simulink model "testBCIRobot3e_sim"  (Simulink 10.0)
settings: Solver=FixedStepDiscrete  StartTime=0.0  StopTime=10  FixedStep=0.002  MaxStep=0.02  RelTol=1e-3  AbsTol=1e-6
libraries: simulink_extras x1
settings Model: Creator=fwornle  LastModifiedBy=bhisma  ExtModeTrigDuration=5000  ExtModeLogAll=off
settings ConfigSet: Description=rtmc9s12target_R2008a
settings SolverCC: AutoScaleAbsTol=off
settings DataIOCC: SignalLoggingSaveFormat=ModelDataLogs  SaveOutput=off  SaveTime=off  SignalLoggingName=sigsOut
settings OptimizationCC: BlockReduction=off  BooleanDataType=off  ExpressionDepthLimit=2147483647  InitFltsAndDblsToZero=on
settings DebuggingCC: SaveWithParameterizedLinksMsg=none  SignalResolutionControl=TryResolveAllWithWarning  MultiTaskDSMMsg=warning  MultiTaskCondExecSysMsg=none  FcnCallInpInsideContextMsg=warning  StateNameClashWarn=warning
settings HardwareCC: ProdBitPerInt=16  ProdBitPerPointer=16  ProdBitPerSizeT=16  ProdBitPerPtrDiffT=16  ProdEndianess=BigEndian  ProdWordSize=16  ProdHWDeviceType=Motorola HC12  TargetHWDeviceType=32-bit Generic  ProdEqTarget=off
settings RTWCC: Description="Visual C/C++ Project Makefile only for the \"grt\" target"  GenerateMakefile=off  TemplateMakefile=grt_msvc.tmf
settings GRTTargetCC: TargetFcnLib=ansi_tfl_tmw.mat  GeneratePreprocessorConditionals=Disable all
settings ConfigComp: CovExternalEMLEnable=off

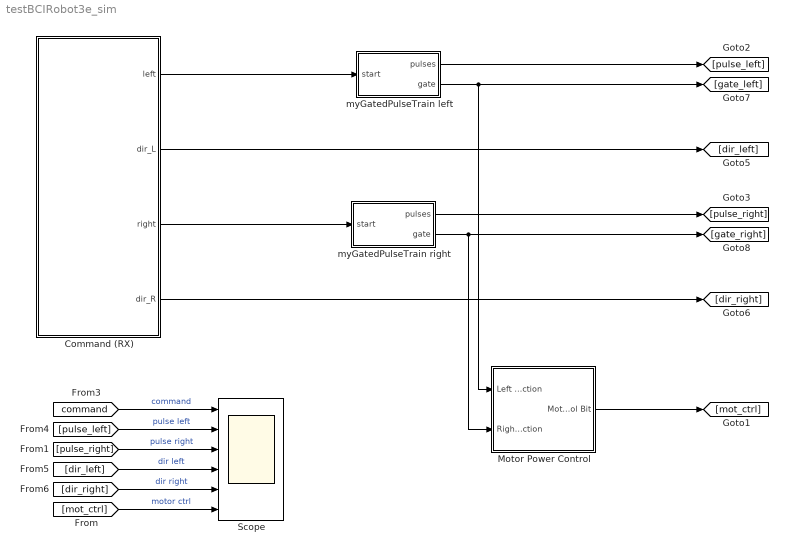
== system testBCIRobot3e_sim ==
  Command (RX) : Subsystem
  Motor Power Control : Subsystem
  Scope : Scope  NumInputPorts=6
  myGatedPulseTrain left : Subsystem  mask{Tcount=0.02, Nsamp=30}
      mask prompts: Tcount "Sample time"; Nsamp "Number of samples"
      mask init:
      | % each period has an on-phase and an off-phase
      | Ncount = 2*Nsamp;
  myGatedPulseTrain right : Subsystem  mask{Tcount=0.02, Nsamp=30}
      mask prompts: Tcount "Sample time"; Nsamp "Number of samples"
      mask init:
      | % each period has an on-phase and an off-phase
      | Ncount = 2*Nsamp;
  wires:
  [command] -> Scope/1  "command"
  [pulse_left] -> Scope/2  "pulse left"
  [pulse_right] -> Scope/3  "pulse right"
  [dir_left] -> Scope/4  "dir left"
  [dir_right] -> Scope/5  "dir right"
  [mot_ctrl] -> Scope/6  "motor ctrl"
  myGatedPulseTrain left/2(gate) -> [gate_left], Motor Power Control/1(Left Motor Instruction)
  myGatedPulseTrain right/2(gate) -> [gate_right], Motor Power Control/2(Right Motor  Instruction)
  myGatedPulseTrain left/1(pulses) -> [pulse_left]
  myGatedPulseTrain right/1(pulses) -> [pulse_right]
  Command (RX)/1(left) -> myGatedPulseTrain left/1(start)
  Command (RX)/3(right) -> myGatedPulseTrain right/1(start)
  Command (RX)/2(dir_L) -> [dir_left]
  Command (RX)/4(dir_R) -> [dir_right]
  Motor Power Control/1(Motor Control Bit) -> [mot_ctrl]

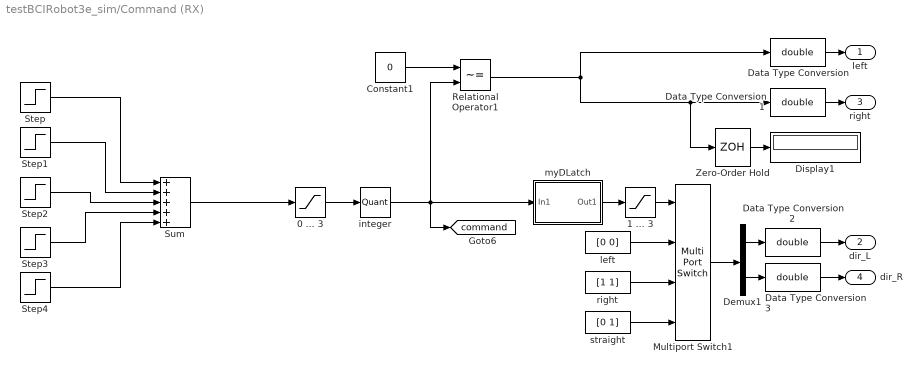
== system testBCIRobot3e_sim/Command (RX) ==
  " left " : Constant  Value=[0 0]  OutDataTypeStr=double
  " right " : Constant  Value=[1 1]  OutDataTypeStr=double
  " straight " : Constant  Value=[0 1]  OutDataTypeStr=double
  0 ... 3 : Saturate  UpperLimit=3  LowerLimit=0  SampleTime=0.002
  1 ... 3 : Saturate  UpperLimit=3  LowerLimit=1
  Constant1 : Constant  Value=0
  Data Type Conversion{,1..3} (4 alike) : DataTypeConversion  OutDataTypeStr=double  SaturateOnIntegerOverflow=on  RndMeth=Zero
  Demux1 : Demux  Outputs=2
  Display1 : Display
  Multiport Switch1 : MultiPortSwitch  SaturateOnIntegerOverflow=on
  Relational Operator1 : RelationalOperator  Operator=~=  OutDataTypeStr=uint(8)  RndMeth=Nearest
  Step : Step  After=3  SampleTime=0
  Step1 : Step  Time=2  After=-2  SampleTime=0
  Step2 : Step  Time=2.1  After=-1  SampleTime=0
  Step3 : Step  Time=4  After=2  SampleTime=0
  Step4 : Step  Time=4.2  After=-2  SampleTime=0
  Sum : Sum  Inputs=+++++  SaturateOnIntegerOverflow=on
  Zero-Order Hold : ZeroOrderHold  SampleTime=0.1
  integer : Quantizer  QuantizationInterval=1
  myDLatch : Subsystem
  left : Outport
  dir_L : Outport  Port=2
  right : Outport  Port=3
  dir_R : Outport  Port=4
  tag scope: command=global
  wires:
  0 ... 3/1 -> integer/1
  " left "/1 -> Multiport Switch1/2
  " right "/1 -> Multiport Switch1/3
  " straight "/1 -> Multiport Switch1/4
  Multiport Switch1/1 -> Demux1/1
  Demux1/1 -> Data Type Conversion2/1
  Demux1/2 -> Data Type Conversion3/1
  1 ... 3/1 -> Multiport Switch1/1
  Data Type Conversion2/1 -> dir_L/1
  Data Type Conversion3/1 -> dir_R/1
  myDLatch/1(Out1) -> 1 ... 3/1
  Sum/1 -> 0 ... 3/1
  integer/1 -> myDLatch/1(In1), [command], Relational Operator1/2
  Step/1 -> Sum/1
  Step1/1 -> Sum/2
  Step2/1 -> Sum/3
  Step3/1 -> Sum/4
  Step4/1 -> Sum/5
  Constant1/1 -> Relational Operator1/1
  Data Type Conversion/1 -> left/1
  Data Type Conversion1/1 -> right/1
  Relational Operator1/1 -> Data Type Conversion/1, Data Type Conversion1/1, Zero-Order Hold/1
  Zero-Order Hold/1 -> Display1/1

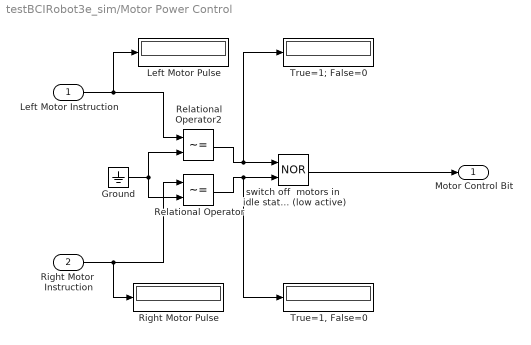
== system testBCIRobot3e_sim/Motor Power Control ==
  Left Motor Instruction : Inport
  Right Motor  Instruction : Inport  Port=2
  Ground : Ground
  Left Motor Pulse : Display
  Relational Operator : RelationalOperator  Operator=~=  RndMeth=Nearest
  Relational Operator2 : RelationalOperator  Operator=~=  RndMeth=Nearest
  Right Motor Pulse : Display
  "True=1, False=0" : Display
  True=1; False=0 : Display
  switch off  motors in  idle state (low active) : Logic  Operator=NOR  AllPortsSameDT=off
  Motor Control Bit : Outport
  wires:
  switch off  motors in  idle state (low active)/1 -> Motor Control Bit/1
  Relational Operator/1 -> "True=1, False=0"/1, switch off  motors in  idle state (low active)/2
  Relational Operator2/1 -> True=1; False=0/1, switch off  motors in  idle state (low active)/1
  Ground/1 -> Relational Operator/2, Relational Operator2/2
  Left Motor Instruction/1 -> Left Motor Pulse/1, Relational Operator2/1
  Right Motor  Instruction/1 -> Right Motor Pulse/1, Relational Operator/1

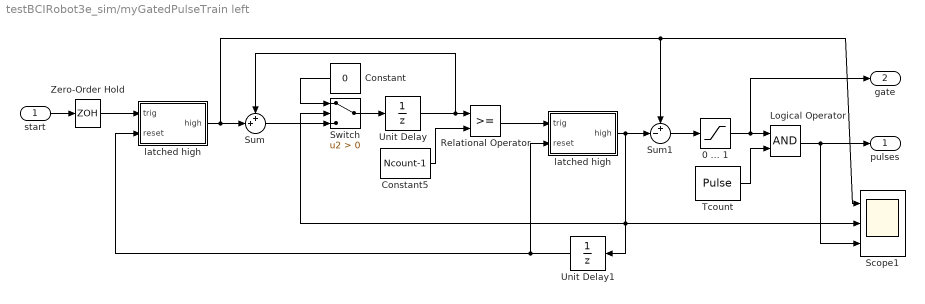
== system testBCIRobot3e_sim/myGatedPulseTrain left ==
  start : Inport
  " latched high " : Subsystem
  0 ... 1 : Saturate  UpperLimit=1  LowerLimit=0
  Constant : Constant  Value=0
  Constant5 : Constant  Value=Ncount-1
  Logical Operator : Logic  AllPortsSameDT=off
  Relational Operator : RelationalOperator  OutDataTypeStr=uint(8)  RndMeth=Nearest
  Scope1 : Scope  NumInputPorts=3
  Sum : Sum  Inputs=++|
  Sum1 : Sum  Inputs=+-|
  Switch : Switch  Criteria=u2 > Threshold
  Tcount : DiscretePulseGenerator  SampleTime=Tcount
  Unit Delay : UnitDelay  SampleTime=Tcount
  Unit Delay1 : UnitDelay  SampleTime=Tcount
  Zero-Order Hold : ZeroOrderHold  SampleTime=Tcount
  latched high : Subsystem
  pulses : Outport
  gate : Outport  Port=2
  wires:
  latched high/1(high) -> Sum/2, Sum1/1, Scope1/1
  start/1 -> Zero-Order Hold/1
  Constant5/1 -> Relational Operator/2
  Constant/1 -> Switch/1
  Sum/1 -> Switch/3
  Unit Delay/1 -> Relational Operator/1, Sum/1
  Switch/1 -> Unit Delay/1
  Sum1/1 -> 0 ... 1/1
  Relational Operator/1 -> " latched high "/1(trig)
  " latched high "/1(high) -> Sum1/2, Scope1/2, Switch/2, Unit Delay1/1
  Unit Delay1/1 -> " latched high "/2(reset), latched high/2(reset)
  0 ... 1/1 -> Logical Operator/1, gate/1
  Tcount/1 -> Logical Operator/2
  Logical Operator/1 -> pulses/1, Scope1/3
  Zero-Order Hold/1 -> latched high/1(trig)

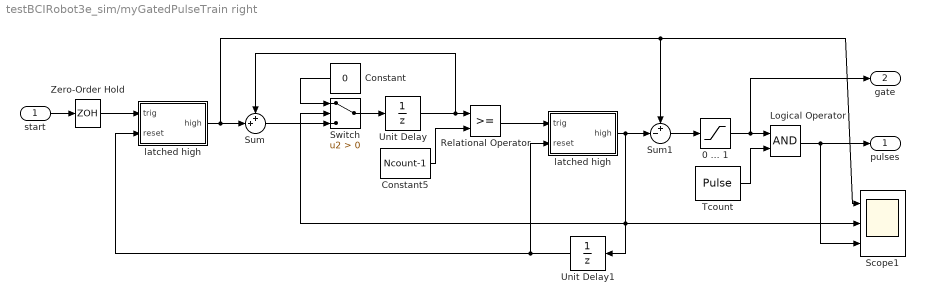
== system testBCIRobot3e_sim/myGatedPulseTrain right ==
  start : Inport
  " latched high " : Subsystem
  0 ... 1 : Saturate  UpperLimit=1  LowerLimit=0
  Constant : Constant  Value=0
  Constant5 : Constant  Value=Ncount-1
  Logical Operator : Logic  AllPortsSameDT=off
  Relational Operator : RelationalOperator  OutDataTypeStr=uint(8)  RndMeth=Nearest
  Scope1 : Scope  NumInputPorts=3
  Sum : Sum  Inputs=++|
  Sum1 : Sum  Inputs=+-|
  Switch : Switch  Criteria=u2 > Threshold
  Tcount : DiscretePulseGenerator  SampleTime=Tcount
  Unit Delay : UnitDelay  SampleTime=Tcount
  Unit Delay1 : UnitDelay  SampleTime=Tcount
  Zero-Order Hold : ZeroOrderHold  SampleTime=Tcount
  latched high : Subsystem
  pulses : Outport
  gate : Outport  Port=2
  wires:
  Zero-Order Hold/1 -> latched high/1(trig)
  Logical Operator/1 -> Scope1/3, pulses/1
  Tcount/1 -> Logical Operator/2
  0 ... 1/1 -> gate/1, Logical Operator/1
  Unit Delay1/1 -> latched high/2(reset), " latched high "/2(reset)
  " latched high "/1(high) -> Unit Delay1/1, Switch/2, Scope1/2, Sum1/2
  Relational Operator/1 -> " latched high "/1(trig)
  Sum1/1 -> 0 ... 1/1
  Switch/1 -> Unit Delay/1
  Unit Delay/1 -> Sum/1, Relational Operator/1
  Sum/1 -> Switch/3
  Constant/1 -> Switch/1
  Constant5/1 -> Relational Operator/2
  start/1 -> Zero-Order Hold/1
  latched high/1(high) -> Scope1/1, Sum1/1, Sum/2

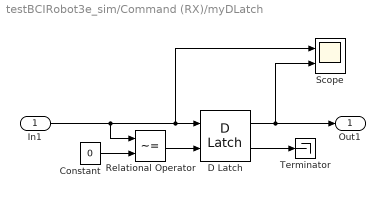
== system testBCIRobot3e_sim/Command (RX)/myDLatch ==
  In1 : Inport
  Constant : Constant  Value=0
  D Latch : simulink_extras/Flip Flops/D Latch  SystemSampleTime=-1
      settings: SourceProductName=Simulink  SourceProductBaseCode=SL
  Relational Operator : RelationalOperator  Operator=~=  RndMeth=Nearest
  Scope : Scope  NumInputPorts=2
  Terminator : Terminator
  Out1 : Outport
  wires:
  D Latch/2 -> Terminator/1
  D Latch/1 -> Out1/1, Scope/2
  In1/1 -> Relational Operator/1, D Latch/1, Scope/1
  Constant/1 -> Relational Operator/2
  Relational Operator/1 -> D Latch/2

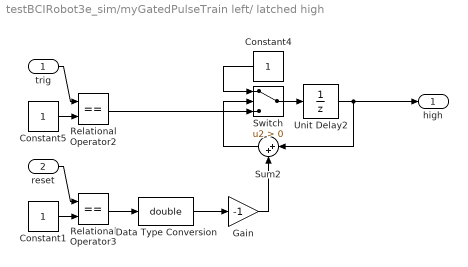
== system testBCIRobot3e_sim/myGatedPulseTrain left/ latched high  ==
  trig : Inport
  reset : Inport  Port=2
  Constant1 : Constant
  Constant4 : Constant
  Constant5 : Constant
  Data Type Conversion : DataTypeConversion  OutDataTypeStr=double  SaturateOnIntegerOverflow=on  RndMeth=Zero
  Gain : Gain  Gain=-1  SaturateOnIntegerOverflow=on  OutDataTypeStr=Inherit: Same as input  ParamDataTypeStr=Inherit: Same as input
  Relational Operator2 : RelationalOperator  Operator===  OutDataTypeStr=uint(8)  RndMeth=Nearest
  Relational Operator3 : RelationalOperator  Operator===  OutDataTypeStr=uint(8)  RndMeth=Nearest
  Sum2 : Sum  Inputs=|++
  Switch : Switch  Criteria=u2 > Threshold
  Unit Delay2 : UnitDelay  SampleTime=-1
  high : Outport
  wires:
  Constant5/1 -> Relational Operator2/2
  Relational Operator2/1 -> Switch/3
  Unit Delay2/1 -> Sum2/1, high/1
  Constant4/1 -> Switch/1
  Switch/1 -> Unit Delay2/1
  Sum2/1 -> Switch/2
  Constant1/1 -> Relational Operator3/2
  Relational Operator3/1 -> Data Type Conversion/1
  Gain/1 -> Sum2/2
  Data Type Conversion/1 -> Gain/1
  reset/1 -> Relational Operator3/1
  trig/1 -> Relational Operator2/1

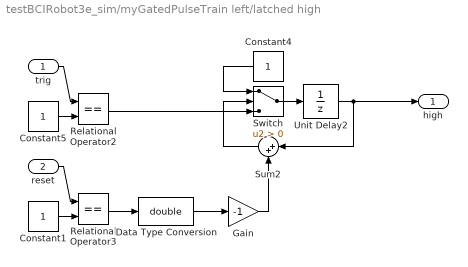
== system testBCIRobot3e_sim/myGatedPulseTrain left/latched high ==
  trig : Inport
  reset : Inport  Port=2
  Constant1 : Constant
  Constant4 : Constant
  Constant5 : Constant
  Data Type Conversion : DataTypeConversion  OutDataTypeStr=double  SaturateOnIntegerOverflow=on  RndMeth=Zero
  Gain : Gain  Gain=-1  SaturateOnIntegerOverflow=on  OutDataTypeStr=Inherit: Same as input  ParamDataTypeStr=Inherit: Same as input
  Relational Operator2 : RelationalOperator  Operator===  OutDataTypeStr=uint(8)  RndMeth=Nearest
  Relational Operator3 : RelationalOperator  Operator===  OutDataTypeStr=uint(8)  RndMeth=Nearest
  Sum2 : Sum  Inputs=|++
  Switch : Switch  Criteria=u2 > Threshold
  Unit Delay2 : UnitDelay  SampleTime=-1
  high : Outport
  wires:
  trig/1 -> Relational Operator2/1
  reset/1 -> Relational Operator3/1
  Data Type Conversion/1 -> Gain/1
  Gain/1 -> Sum2/2
  Relational Operator3/1 -> Data Type Conversion/1
  Constant1/1 -> Relational Operator3/2
  Sum2/1 -> Switch/2
  Switch/1 -> Unit Delay2/1
  Constant4/1 -> Switch/1
  Unit Delay2/1 -> high/1, Sum2/1
  Relational Operator2/1 -> Switch/3
  Constant5/1 -> Relational Operator2/2

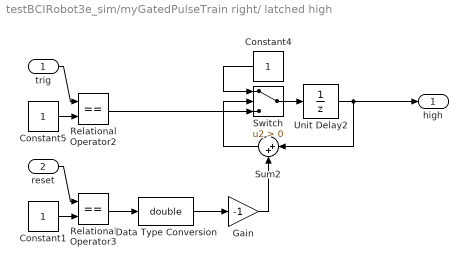
== system testBCIRobot3e_sim/myGatedPulseTrain right/ latched high  ==
  trig : Inport
  reset : Inport  Port=2
  Constant1 : Constant
  Constant4 : Constant
  Constant5 : Constant
  Data Type Conversion : DataTypeConversion  OutDataTypeStr=double  SaturateOnIntegerOverflow=on  RndMeth=Zero
  Gain : Gain  Gain=-1  SaturateOnIntegerOverflow=on  OutDataTypeStr=Inherit: Same as input  ParamDataTypeStr=Inherit: Same as input
  Relational Operator2 : RelationalOperator  Operator===  OutDataTypeStr=uint(8)  RndMeth=Nearest
  Relational Operator3 : RelationalOperator  Operator===  OutDataTypeStr=uint(8)  RndMeth=Nearest
  Sum2 : Sum  Inputs=|++
  Switch : Switch  Criteria=u2 > Threshold
  Unit Delay2 : UnitDelay  SampleTime=-1
  high : Outport
  wires:
  trig/1 -> Relational Operator2/1
  reset/1 -> Relational Operator3/1
  Data Type Conversion/1 -> Gain/1
  Gain/1 -> Sum2/2
  Relational Operator3/1 -> Data Type Conversion/1
  Constant1/1 -> Relational Operator3/2
  Sum2/1 -> Switch/2
  Switch/1 -> Unit Delay2/1
  Constant4/1 -> Switch/1
  Unit Delay2/1 -> high/1, Sum2/1
  Relational Operator2/1 -> Switch/3
  Constant5/1 -> Relational Operator2/2

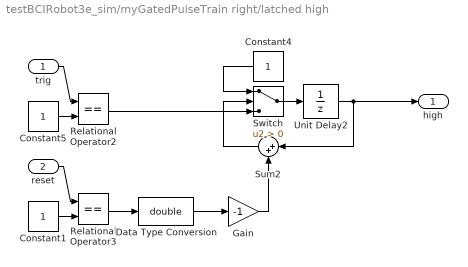
== system testBCIRobot3e_sim/myGatedPulseTrain right/latched high ==
  trig : Inport
  reset : Inport  Port=2
  Constant1 : Constant
  Constant4 : Constant
  Constant5 : Constant
  Data Type Conversion : DataTypeConversion  OutDataTypeStr=double  SaturateOnIntegerOverflow=on  RndMeth=Zero
  Gain : Gain  Gain=-1  SaturateOnIntegerOverflow=on  OutDataTypeStr=Inherit: Same as input  ParamDataTypeStr=Inherit: Same as input
  Relational Operator2 : RelationalOperator  Operator===  OutDataTypeStr=uint(8)  RndMeth=Nearest
  Relational Operator3 : RelationalOperator  Operator===  OutDataTypeStr=uint(8)  RndMeth=Nearest
  Sum2 : Sum  Inputs=|++
  Switch : Switch  Criteria=u2 > Threshold
  Unit Delay2 : UnitDelay  SampleTime=-1
  high : Outport
  wires:
  Constant5/1 -> Relational Operator2/2
  Relational Operator2/1 -> Switch/3
  Unit Delay2/1 -> Sum2/1, high/1
  Constant4/1 -> Switch/1
  Switch/1 -> Unit Delay2/1
  Sum2/1 -> Switch/2
  Constant1/1 -> Relational Operator3/2
  Relational Operator3/1 -> Data Type Conversion/1
  Gain/1 -> Sum2/2
  Data Type Conversion/1 -> Gain/1
  reset/1 -> Relational Operator3/1
  trig/1 -> Relational Operator2/1
